simulink model "L0708"  (Simulink 10.2)
settings: Solver=VariableStepDiscrete  StartTime=0.0  StopTime=10  MaxStep=0.01  RelTol=1e-3
InitFcn:
  | data3
values from neighbouring files (symbols this model uses):
  Alpha = 65    [data1.m]    (also in data3.m)
  g = 9.81    [data.m]
  L = 15    [data.m]    (also in data3.m = 10)
  V0 = 17    [data1.m]    (also in data3.m)
  x0 = []    [L0706Plot.m]    (also in L0708Plot.m; data.m = 1)
  y0 = 5    [data.m]
libraries: simulink x2
settings Model: Creator=Ranci  LastModifiedBy=Ranci
settings DataIOCC: SaveFormat=Dataset  SignalLoggingSaveFormat=Dataset  ReturnWorkspaceOutputs=on
settings OptimizationCC: LifeSpan=auto
settings DebuggingCC: UnderspecifiedInitializationDetection=Simplified  MergeDetectMultiDrivingBlocksExec=error  FcnCallInpInsideContextMsg=error  SFUnexpectedBacktrackingDiag=error  SFNoUnconditionalDefaultTransitionDiag=error  SFExecutionAtInitializationDiag=warning  ArithmeticOperatorsInVariantConditions=error
settings HardwareCC: ProdBitPerPointer=64  ProdBitPerSizeT=64  ProdBitPerPtrDiffT=64  ProdLargestAtomicFloat=Float  ProdIntDivRoundTo=Zero  ProdEndianess=LittleEndian  ProdWordSize=64  ProdHWDeviceType=Intel->x86-64 (Windows64)
settings ModelReferenceCC: PropagateSignalLabelsOutOfModel=on
settings SFSimCC: SimUseLocalCustomCode=on  CustomCodeUndefinedFunction=FilterOut
settings RTWCC: RTWUseLocalCustomCode=on
settings CodeAppCC: StateflowObjectComments=off
settings GRTTargetCC: TargetLangStandard=C99 (ISO)  CombineOutputUpdateFcns=on  GRTInterface=off
settings ConfigComp: CovMetricSettings=dwe  CovSaveCumulativeToWorkspaceVar=off  CovSaveSingleToWorkspaceVar=off  CovExternalEMLEnable=on

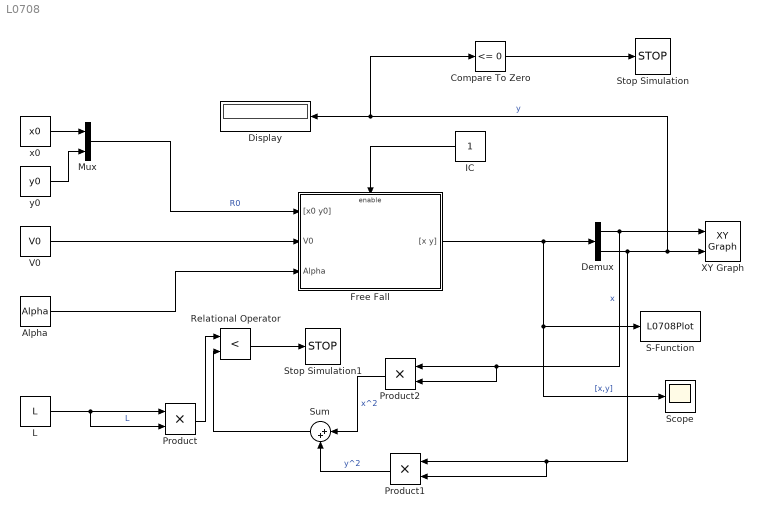
== system L0708 ==
  Alpha : Constant  Value=Alpha
  Compare To Zero : simulink/Logic and Bit Operations/Compare To Zero  relop=<=  OutDataTypeStr=boolean
  Demux : Demux  Outputs=2
  Display : Display
  Free Fall : Subsystem  TreatAsAtomicUnit=on
  IC : Constant
  L : Constant  Value=L
  Mux : Mux  Inputs=2
  Product : Product
  Product1 : Product
  Product2 : Product
  Relational Operator : RelationalOperator  Operator=<  OutDataTypeStr=boolean  RndMeth=Simplest
  S-Function : S-Function  FunctionName=L0708Plot  Parameters=0.1,x0,y0  SFunctionDeploymentMode=off  EnableBusSupport=off
  Scope : Scope
  Stop Simulation : Stop
  Stop Simulation1 : Stop
  Sum : Sum  Inputs=|++
  V0 : Constant  Value=V0
  XY Graph : simulink/Sinks/XY Graph  xmin=0  xmax=30  ymin=0  ymax=20  st=-1
  x0 : Constant  Value=x0
  y0 : Constant  Value=y0
  wires:
  x0/1 -> Mux/1
  y0/1 -> Mux/2
  Mux/1 -> Free Fall/1("[x0 y0]")  "R0"
  Free Fall/1("[x y]") -> S-Function/1, Scope/1, Demux/1  "[x,y]"
  Demux/1 -> Product2/2, Product2/1, XY Graph/1  "x"
  Demux/2 -> Product1/2, Product1/1, Compare To Zero/1, Display/1, XY Graph/2  "y"
  Compare To Zero/1 -> Stop Simulation/1
  IC/1 -> Free Fall/Enable
  V0/1 -> Free Fall/2(V0)
  Alpha/1 -> Free Fall/3(Alpha)
  L/1 -> Product/2, Product/1  "L"
  Product2/1 -> Sum/1  "x^2"
  Product1/1 -> Sum/2  "y^2"
  Product/1 -> Relational Operator/1
  Sum/1 -> Relational Operator/2
  Relational Operator/1 -> Stop Simulation1/1

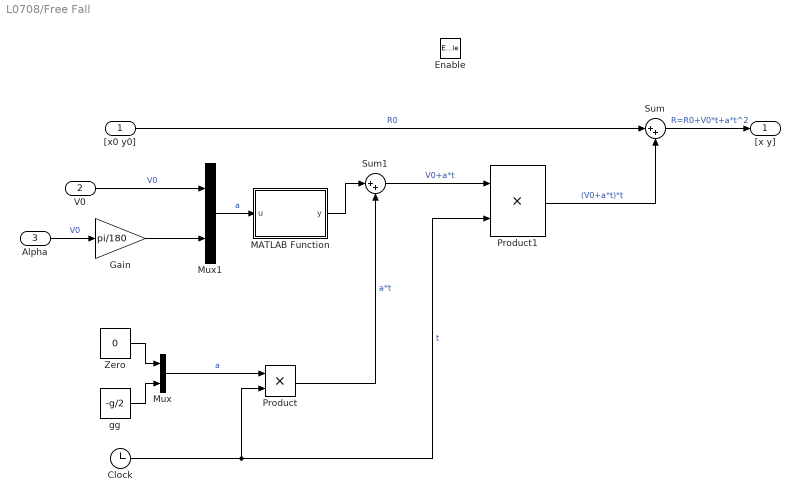
== system L0708/Free Fall ==
  "[x0 y0]" : Inport
  V0 : Inport  Port=2
  Alpha : Inport  Port=3
  Enable : EnablePort
  Clock : Clock
  Gain : Gain  Gain=pi/180
  MATLAB Function : MATLAB Function  TreatAsAtomicUnit=on
  Mux : Mux  Inputs=2
  Mux1 : Mux  Inputs=2
  Product : Product
  Product1 : Product
  Sum : Sum  Inputs=|++
  Sum1 : Sum  Inputs=|++
  Zero : Constant  Value=0
  gg : Constant  Value=-g/2
  "[x y]" : Outport
  wires:
  "[x0 y0]"/1 -> Sum/1  "R0"
  gg/1 -> Mux/2
  Zero/1 -> Mux/1
  Mux/1 -> Product/1  "a"
  Clock/1 -> Product1/2, Product/2  "t"
  Product/1 -> Sum1/2  "a*t"
  Sum1/1 -> Product1/1  "V0+a*t"
  Product1/1 -> Sum/2  "(V0+a*t)*t"
  Sum/1 -> "[x y]"/1  "R=R0+V0*t+a*t^2"
  Alpha/1 -> Gain/1  "V0"
  Gain/1 -> Mux1/2
  V0/1 -> Mux1/1  "V0"
  Mux1/1 -> MATLAB Function/1(u)  "a"
  MATLAB Function/1(y) -> Sum1/1

== matlab function Free Fall/MATLAB Function ==
  data: u input double; y output double
function y = fcn(u)
Vx0 = u(1) * cos(u(2));
Vy0 = u(1) * sin(u(2));
y = [Vx0 Vy0];
